simulink model "m03_linearization_model_4DOF"  (R2021a)
settings: Solver=VariableStepAuto  StartTime=0.0  StopTime=10  RelTol=1e-3
values from neighbouring files (symbols this model uses):
  a = L - b    (= 1.43208)    [m00_params.m]    (also in params.mat)
  b = distr*L/(1 + distr)    (= 1.62792)    [m00_params.m]    (also in params.mat)
  F_damper = [-2018 -1498 -1198 -898 -530 0 305 552 734 942 1306]    [damper.mat]    (also in m00_params.m = F_damper)
  Ff_spring = [-4676.870968 -4635.060192 -4593.2364576 -4551.3997648 -4509.5501136 -4467.687504 -4425.811936 -4383.9234096 -4342.0219248 -4300.1074816 -4258.18008 -4216.23972 ... (221 elements, 1x221)]    [spring.mat]
  Fr_spring = [-6174.79580863 -6119.36435311 -6063.92211228 -6008.46902741 -5953.00503974 -5897.53009054 -5842.04412106 -5786.54707256 -5731.0388863 -5675.51950353 -5619.98886552 -5564.44691352 ... (221 elements, 1x221)]    [spring.mat]
  FzF_0_w = FzF_0/2    (= 6523.65)    [m00_params.m]
  FzR_0_w = FzR_0/2    (= 5738.85)    [m00_params.m]
  h_CoG = 0.642    [m00_params.m]    (also in params.mat)
  h_RC = h_CoG - hs    (= 0.116)    [m00_params.m]    (also in params2.mat)
  hs = 0.526    [m00_params.m]
  hu = 0.4    [m00_params.m]    (also in params2.mat)
  Ix = 850    [m00_params.m]
  Iz = 4600    [m00_params.m]
  Kt = (Kt_f + Kt_r)/2    (= 306000)    [m00_params.m]
  M = 2500    [m00_params.m]    (also in params.mat)
  ms = M - mu    (= 2159)    [m00_params.m]
  mu = 2*(mui)    (= 341)    [m00_params.m]
  mui = mui_f + mui_r    (= 170.5)    [m00_params.m]
  tw = (tw_F + tw_R)/2    (= 1.6675)    [m00_params.m]
  v_damper = [-0.52 -0.26 -0.13 -0.05 -0.02 0 0.02 0.05 0.13 0.26 0.52]    [damper.mat]
  Z_spring = [-0.11 -0.109 -0.108 -0.107 -0.106 -0.105 -0.104 -0.103 -0.102 -0.101 -0.1 -0.099 ... (221 elements, 1x221)]    [spring.mat]
settings Model: Creator=jaime  LastModifiedBy=jaime

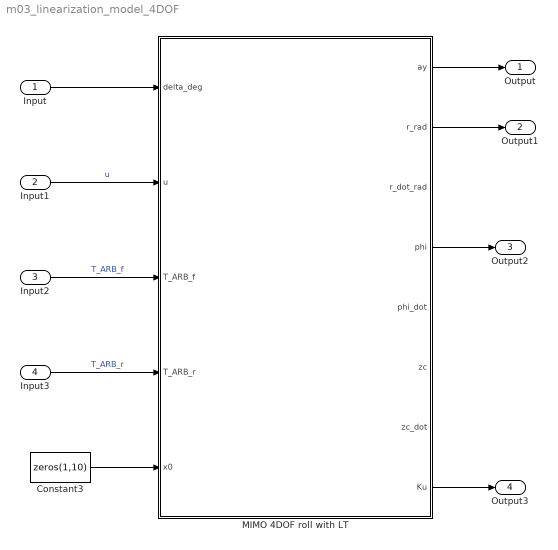
== system m03_linearization_model_4DOF ==
  Input : Inport
  Input1 : Inport  Port=2
  Input2 : Inport  Port=3
  Input3 : Inport  Port=4
  Constant3 : Constant  Value=zeros(1,10)
  MIMO 4DOF roll with LT : Subsystem
  Output : Outport
  Output1 : Outport  Port=2
  Output2 : Outport  Port=3
  Output3 : Outport  Port=4
  wires:
  Input1/1 -> MIMO 4DOF roll with LT/2(u)  "u"
  Input/1 -> MIMO 4DOF roll with LT/1(delta_deg)
  Input2/1 -> MIMO 4DOF roll with LT/3(T_ARB_f)  "T_ARB_f"
  Input3/1 -> MIMO 4DOF roll with LT/4(T_ARB_r)  "T_ARB_r"
  Constant3/1 -> MIMO 4DOF roll with LT/5(x0)
  MIMO 4DOF roll with LT/1(ay) -> Output/1
  MIMO 4DOF roll with LT/2(r_rad) -> Output1/1
  MIMO 4DOF roll with LT/4(phi) -> Output2/1
  MIMO 4DOF roll with LT/8(Ku) -> Output3/1

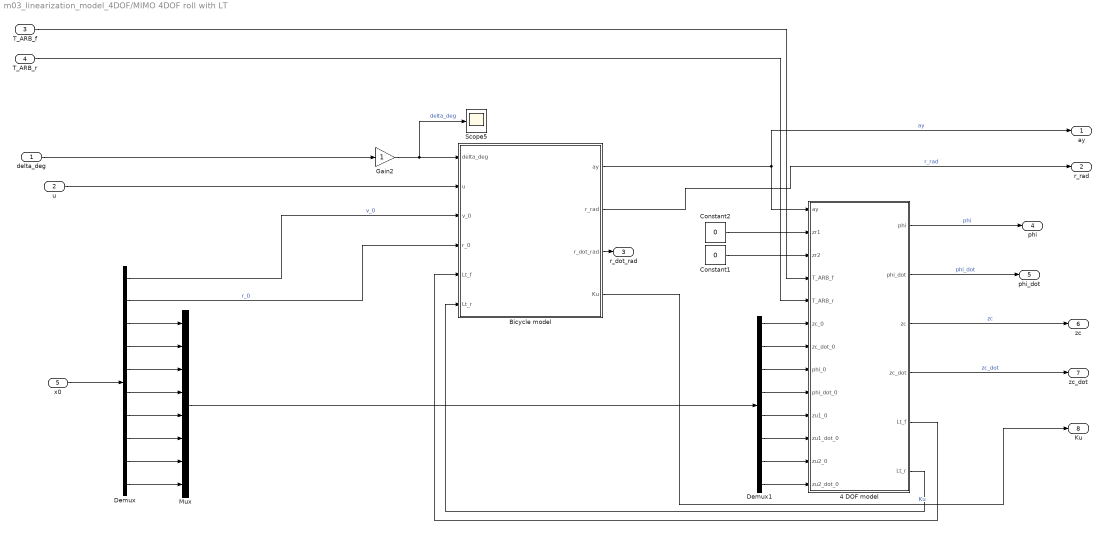
== system m03_linearization_model_4DOF/MIMO 4DOF roll with LT ==
  delta_deg : Inport
  u : Inport  Port=2
  T_ARB_f : Inport  Port=3
  T_ARB_r : Inport  Port=4
  x0 : Inport  Port=5
  4 DOF model : Subsystem
  Bicycle model : Subsystem
  Constant1 : Constant  Value=0
  Constant2 : Constant  Value=0
  Demux : Demux  Outputs=10
  Demux1 : Demux  Outputs=8
  Gain2 : Gain
  Mux : Mux  Inputs=8
  Scope5 : Scope
  ay : Outport
  r_rad : Outport  Port=2
  r_dot_rad : Outport  Port=3
  phi : Outport  Port=4
  phi_dot : Outport  Port=5
  zc : Outport  Port=6
  zc_dot : Outport  Port=7
  Ku : Outport  Port=8
  wires:
  Demux/10 -> Mux/8
  Demux1/6 -> 4 DOF model/11(zu1_dot_0)
  u/1 -> Bicycle model/2(u)
  Gain2/1 -> Scope5/1, Bicycle model/1(delta_deg)  "delta_deg"
  Demux/6 -> Mux/4
  Demux1/8 -> 4 DOF model/13(zu2_dot_0)
  4 DOF model/6(Lt_r) -> Bicycle model/6(Lt_r)
  Demux1/7 -> 4 DOF model/12(zu2_0)
  Demux1/5 -> 4 DOF model/10(zu1_0)
  Demux1/3 -> 4 DOF model/8(phi_0)
  Bicycle model/3(r_dot_rad) -> r_dot_rad/1
  T_ARB_r/1 -> 4 DOF model/5(T_ARB_r)
  Demux/9 -> Mux/7
  Constant1/1 -> 4 DOF model/3(zr2)
  Constant2/1 -> 4 DOF model/2(zr1)
  delta_deg/1 -> Gain2/1
  Bicycle model/1(ay) -> ay/1, 4 DOF model/1(ay)  "ay"
  Demux/3 -> Mux/1
  Demux/5 -> Mux/3
  Mux/1 -> Demux1/1
  Demux1/2 -> 4 DOF model/7(zc_dot_0)
  Demux/7 -> Mux/5
  Bicycle model/4(Ku) -> Ku/1  "Ku"
  4 DOF model/2(phi_dot) -> phi_dot/1  "phi_dot"
  4 DOF model/5(Lt_f) -> Bicycle model/5(Lt_f)
  Demux/4 -> Mux/2
  Demux1/1 -> 4 DOF model/6(zc_0)
  Demux1/4 -> 4 DOF model/9(phi_dot_0)
  Demux/2 -> Bicycle model/4(r_0)  "r_0"
  Demux/8 -> Mux/6
  Demux/1 -> Bicycle model/3(v_0)  "v_0"
  Bicycle model/2(r_rad) -> r_rad/1  "r_rad"
  x0/1 -> Demux/1
  4 DOF model/4(zc_dot) -> zc_dot/1  "zc_dot"
  T_ARB_f/1 -> 4 DOF model/4(T_ARB_f)
  4 DOF model/3(zc) -> zc/1  "zc"
  4 DOF model/1(phi) -> phi/1  "phi"

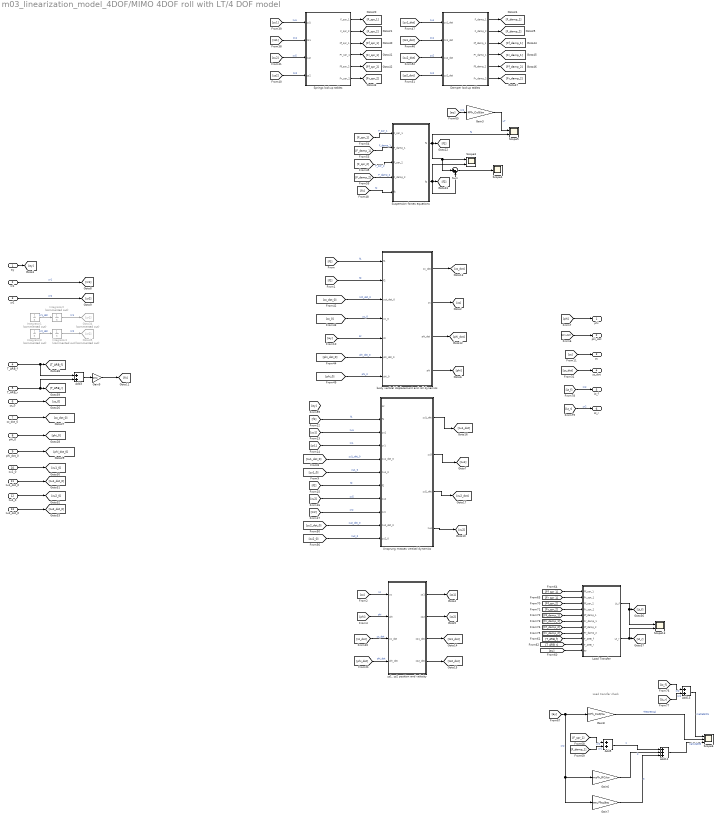
== system m03_linearization_model_4DOF/MIMO 4DOF roll with LT/4 DOF model ==
  note: Load transfer check
  ay : Inport
  zr1 : Inport  Port=2
  zr2 : Inport  Port=3
  T_ARB_f : Inport  Port=4
  T_ARB_r : Inport  Port=5
  zc_0 : Inport  Port=6
  zc_dot_0 : Inport  Port=7
  phi_0 : Inport  Port=8
  phi_dot_0 : Inport  Port=9
  zu1_0 : Inport  Port=10
  zu1_dot_0 : Inport  Port=11
  zu2_0 : Inport  Port=12
  zu2_dot_0 : Inport  Port=13
  Add12 : Sum  Inputs=+++
  Add13 : Sum
  Add3 : Sum
  Add5 : Sum
  Damper lookup tables : Subsystem
  Gain3 : Gain  Gain=M*h_CoG/tw
  Gain6 : Gain  Gain=ms*h_RC/tw
  Gain7 : Gain  Gain=mu*hu/tw
  Gain8 : Gain  Gain=M*h_CoG/tw
  Gain9 : Gain  Gain=1/tw
  Goto34 : Goto  Commented=on  GotoTag=zr1
  Goto35 : Goto  Commented=on  GotoTag=zr2
  Integrator{1..4} (4 alike) : Integrator  Commented=on
  Load Transfer : MATLAB Function  TreatAsAtomicUnit=on
  Scope13 : Scope  NumInputPorts=2
  Scope3 : Scope  NumInputPorts=2
  Scope4 : Scope
  Scope5 : Scope  NumInputPorts=2
  Scope6 : Scope  NumInputPorts=3
  Springs lookup tables : Subsystem
  Sum : Sum  Inputs=|++
  Suspension forces equations : Subsystem
  Unsprung masses vertical dynamics : Subsystem
  body vertical displacement and roll dynamics : Subsystem
  "zs1, zs2 position and velocity" : Subsystem
  phi : Outport
  phi_dot : Outport  Port=2
  zc : Outport  Port=3
  zc_dot : Outport  Port=4
  Lt_f : Outport  Port=5
  Lt_r : Outport  Port=6
  wires:
  [phi] -> phi/1
  ay/1 -> [ay]
  [zc] -> zc/1
  zr1/1 -> [zr1]  "zr1"
  zr2/1 -> [zr2]  "zr2"
  [phi_dot] -> phi_dot/1
  [zc_dot] -> zc_dot/1
  [zu1] -> Springs lookup tables/1(zu1)  "zu1"
  [zs1] -> Springs lookup tables/2(zs1)  "zs1"
  [zu2] -> Springs lookup tables/3(zu2)  "zu2"
  [zs2] -> Springs lookup tables/4(zs2)  "zs2"
  Springs lookup tables/1(F_spr_1) -> [F_spr_1]
  Springs lookup tables/2(F_spr_2) -> [F_spr_2]
  [zu1_dot] -> Damper lookup tables/1(zu1_dot)  "zu1"
  [zs2_dot] -> Damper lookup tables/4(zs2_dot)  "zs2"
  [zs1_dot] -> Damper lookup tables/2(zs1_dot)  "zs1"
  [zu2_dot] -> Damper lookup tables/3(zu2_dot)  "zu2"
  Damper lookup tables/1(F_damp_1) -> [F_damp_1]
  Damper lookup tables/2(F_damp_2) -> [F_damp_2]
  [F_spr_1] -> Suspension forces equations/1(F_spr_1)  "F_spr_1"
  [F_damp_1] -> Suspension forces equations/2(F_damp_1)  "F_damp_1"
  [F_spr_2] -> Suspension forces equations/3(F_spr_2)  "F_spr_2"
  [F_damp_2] -> Suspension forces equations/4(F_damp_2)  "F_damp_2"
  [fc] -> Suspension forces equations/5(fc)  "fc"
  Suspension forces equations/1(f1) -> Scope5/2, [f1], Sum/1, Scope3/1  "f1"
  Suspension forces equations/2(f2) -> Scope3/2, Sum/2, [f2]
  zc_0/1 -> [zc_0]
  zc_dot_0/1 -> [zc_dot_0]
  phi_dot_0/1 -> [phi_dot_0]
  phi_0/1 -> [phi_0]
  [f1] -> body vertical displacement and roll dynamics/1(f1)  "f1"
  [f2] -> body vertical displacement and roll dynamics/2(f2)  "f2"
  [zc_dot_0] -> body vertical displacement and roll dynamics/3(zct_dot_0)  "zct_dot_0"
  [zc_0] -> body vertical displacement and roll dynamics/4(zc_0)  "zc_0"
  [ay] -> body vertical displacement and roll dynamics/5(ay)  "ay"
  [phi_dot_0] -> body vertical displacement and roll dynamics/6(phi_dot_0)  "phi_dot_0"
  [phi_0] -> body vertical displacement and roll dynamics/7(phi_0)  "phi_0"
  body vertical displacement and roll dynamics/1(zc_dot) -> [zc_dot]
  body vertical displacement and roll dynamics/2(zc) -> [zc]
  body vertical displacement and roll dynamics/3(phi_dot) -> [phi_dot]
  body vertical displacement and roll dynamics/4(phi) -> [phi]
  zu1_0/1 -> [zu1_0]
  zu2_dot_0/1 -> [zu2_dot_0]
  zu2_0/1 -> [zu2_0]
  zu1_dot_0/1 -> [zu1_dot_0]
  [f1] -> Unsprung masses vertical dynamics/2(f1)  "f1"
  [zu1] -> Unsprung masses vertical dynamics/3(zu1)  "zu1"
  [zr1] -> Unsprung masses vertical dynamics/4(zr1)  "zr1"
  [zu1_dot_0] -> Unsprung masses vertical dynamics/5(zu1_dot_0)  "zu1_dot_0"
  [zu1_0] -> Unsprung masses vertical dynamics/6(zu1_0)  "zu1_0"
  [f2] -> Unsprung masses vertical dynamics/7(f2)  "f2"
  [zu2] -> Unsprung masses vertical dynamics/8(zu2)  "zu2"
  [zr2] -> Unsprung masses vertical dynamics/9(zr2)  "zr2"
  [zu2_dot_0] -> Unsprung masses vertical dynamics/10(zu2_dot_0)  "zu2_dot_0"
  [zu2_0] -> Unsprung masses vertical dynamics/11(zu2_0)  "zu2_0"
  Unsprung masses vertical dynamics/1(zu1_dot) -> [zu1_dot]
  Unsprung masses vertical dynamics/2(zu3) -> [zu1]
  Unsprung masses vertical dynamics/3(zu2_dot) -> [zu2_dot]
  Unsprung masses vertical dynamics/4(zu4) -> [zu2]
  [zc] -> "zs1, zs2 position and velocity"/1(zc)  "zc"
  [phi] -> "zs1, zs2 position and velocity"/2(phi)  "phi"
  [zc_dot] -> "zs1, zs2 position and velocity"/3(zc_dot)  "zc_dot"
  [phi_dot] -> "zs1, zs2 position and velocity"/4(phi_dot)  "phi_dot"
  "zs1, zs2 position and velocity"/1(zs1) -> [zs1]
  "zs1, zs2 position and velocity"/2(zs2) -> [zs2]
  "zs1, zs2 position and velocity"/3(zs1_dot) -> [zs1_dot]
  "zs1, zs2 position and velocity"/4(zs2_dot) -> [zs2_dot]
  Integrator2/1 -> Goto34/1  "zr1"
  Integrator4/1 -> Goto35/1  "zr2"
  Integrator3/1 -> Integrator4/1  "zr2_dot"
  Integrator1/1 -> Integrator2/1  "zr1_dot"
  Gain9/1 -> [fc]
  T_ARB_f/1 -> Add3/1, [T_ARB_f]
  T_ARB_r/1 -> Add3/2, [T_ARB_r]
  Add3/1 -> Gain9/1
  Sum/1 -> Scope4/1
  [ay] -> Gain3/1  "zr2"
  Gain3/1 -> Scope5/1  "LT"
  Springs lookup tables/3(Ff_spr_1) -> [Ff_spr_1]
  Springs lookup tables/4(Fr_spr_1) -> [Fr_spr_1]
  Springs lookup tables/5(Ff_spr_2) -> [Ff_spr_2]
  Springs lookup tables/6(Fr_spr_2) -> [Fr_spr_2]
  [F_spr_1] -> Add5/1  "zr2"
  [F_damp_1] -> Add5/2  "zr2"
  Add5/1 -> Add12/1  "1"
  [ay] -> Gain8/1, Gain7/1, Gain6/1  "zr2"
  Gain6/1 -> Add12/2  "2"
  Gain7/1 -> Add12/3  "3"
  Add12/1 -> Scope6/3  "calculated"
  Gain8/1 -> Scope6/2  "Theoretical"
  [Ff_spr_1] -> Load Transfer/1(Ff_spr_1)
  [T_ARB_r] -> Load Transfer/10(T_ARB_r)
  [Fr_spr_1] -> Load Transfer/2(Fr_spr_1)
  [T_ARB_f] -> Load Transfer/9(T_ARB_f)
  Load Transfer/1(Lt_f) -> Scope13/1, [Lt_f]
  [ay] -> Load Transfer/11(ay)
  Load Transfer/2(Lt_r) -> Scope13/2, [Lt_r]
  Damper lookup tables/3(Ff_damp_1) -> [Ff_damp_1]
  Damper lookup tables/4(Fr_damp_1) -> [Fr_damp_1]
  Damper lookup tables/5(Ff_damp_2) -> [Ff_damp_2]
  Damper lookup tables/6(Fr_damp_2) -> [Fr_damp_2]
  [Ff_spr_2] -> Load Transfer/3(Ff_spr_2)
  [Fr_spr_2] -> Load Transfer/4(Fr_spr_2)
  [Ff_damp_1] -> Load Transfer/5(Ff_damp_1)
  [Fr_damp_1] -> Load Transfer/6(Fr_damp_1)
  [Ff_damp_2] -> Load Transfer/7(Ff_damp_2)
  [Fr_damp_2] -> Load Transfer/8(Fr_damp_2)
  [Lt_f] -> Add13/1  "zr2"
  [Lt_r] -> Add13/2  "zr2"
  Add13/1 -> Scope6/1  "matlabFCN"
  [Lt_f] -> Lt_f/1  "zr2"
  [Lt_r] -> Lt_r/1  "zr2"

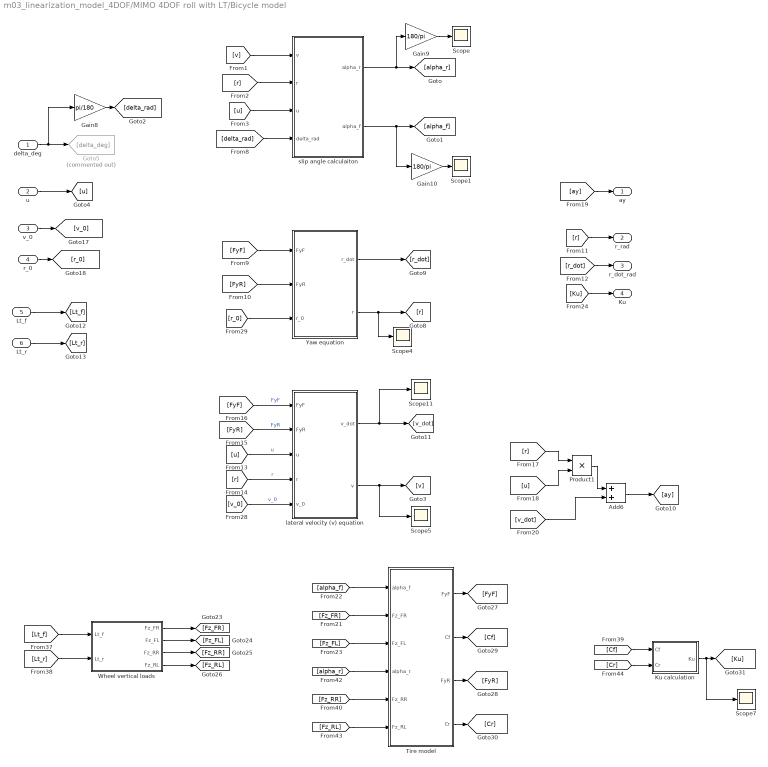
== system m03_linearization_model_4DOF/MIMO 4DOF roll with LT/Bicycle model ==
  delta_deg : Inport
  u : Inport  Port=2
  v_0 : Inport  Port=3
  r_0 : Inport  Port=4
  Lt_f : Inport  Port=5
  Lt_r : Inport  Port=6
  Add6 : Sum
  Gain10 : Gain  Gain=180/pi
  Gain8 : Gain  Gain=pi/180
  Gain9 : Gain  Gain=180/pi
  Goto5 : Goto  Commented=on  GotoTag=delta_deg
  Ku calculation : MATLAB Function  TreatAsAtomicUnit=on
  Product1 : Product
  Scope{,1,4..5,7,11} (6 alike) : Scope
  Tire model : Subsystem
      settings: AttributesFormatString=%<MinAlgLoopOccurrences>
  Wheel vertical loads : Subsystem
      settings: AttributesFormatString=%<MinAlgLoopOccurrences>
  Yaw equation : Subsystem
  lateral velocity (v) equation : Subsystem
  slip angle calculaiton : Subsystem
  ay : Outport
  r_rad : Outport  Port=2
  r_dot_rad : Outport  Port=3
  Ku : Outport  Port=4
  wires:
  u/1 -> [u]
  delta_deg/1 -> Gain8/1, Goto5/1
  [r] -> r_rad/1
  [r_dot] -> r_dot_rad/1
  [r] -> Product1/1
  [u] -> Product1/2
  [ay] -> ay/1
  Gain8/1 -> [delta_rad]
  Add6/1 -> [ay]
  Product1/1 -> Add6/1
  [v_dot] -> Add6/2
  Wheel vertical loads/4(Fz_RL) -> [Fz_RL]
  [Lt_f] -> Wheel vertical loads/1(Lt_f)
  [Lt_r] -> Wheel vertical loads/2(Lt_r)
  Wheel vertical loads/1(Fz_FR) -> [Fz_FR]
  Wheel vertical loads/3(Fz_RR) -> [Fz_RR]
  Wheel vertical loads/2(Fz_FL) -> [Fz_FL]
  Lt_f/1 -> [Lt_f]
  Lt_r/1 -> [Lt_r]
  [Fz_RR] -> Tire model/5(Fz_RR)
  Tire model/3(FyR) -> [FyR]
  Tire model/2(Cf) -> [Cf]
  Tire model/1(FyF) -> [FyF]
  [Fz_FL] -> Tire model/3(Fz_FL)
  [Fz_FR] -> Tire model/2(Fz_FR)
  [alpha_r] -> Tire model/4(alpha_r)
  Tire model/4(Cr) -> [Cr]
  [Fz_RL] -> Tire model/6(Fz_RL)
  [alpha_f] -> Tire model/1(alpha_f)
  [Cr] -> Ku calculation/2(Cr)
  [Cf] -> Ku calculation/1(Cf)
  Ku calculation/1(Ku) -> Scope7/1, [Ku]
  [Ku] -> Ku/1
  slip angle calculaiton/2(alpha_f) -> Gain10/1, [alpha_f]
  [r] -> slip angle calculaiton/2(r)
  [u] -> slip angle calculaiton/3(u)
  slip angle calculaiton/1(alpha_r) -> [alpha_r], Gain9/1
  Gain9/1 -> Scope/1
  [delta_rad] -> slip angle calculaiton/4(delta_rad)
  Gain10/1 -> Scope1/1
  [v] -> slip angle calculaiton/1(v)
  v_0/1 -> [v_0]
  r_0/1 -> [r_0]
  [r_0] -> Yaw equation/3(r_0)
  [FyR] -> Yaw equation/2(FyR)
  Yaw equation/1(r_dot) -> [r_dot]
  [FyF] -> Yaw equation/1(FyF)
  Yaw equation/2(r) -> [r], Scope4/1
  [FyR] -> lateral velocity (v) equation/2(FyR)  "FyR"
  [u] -> lateral velocity (v) equation/3(u)  "u"
  [FyF] -> lateral velocity (v) equation/1(FyF)  "FyF"
  [v_0] -> lateral velocity (v) equation/5(v_0)  "v_0"
  lateral velocity (v) equation/2(v) -> [v], Scope5/1
  lateral velocity (v) equation/1(v_dot) -> [v_dot], Scope11/1
  [r] -> lateral velocity (v) equation/4(r)  "r"

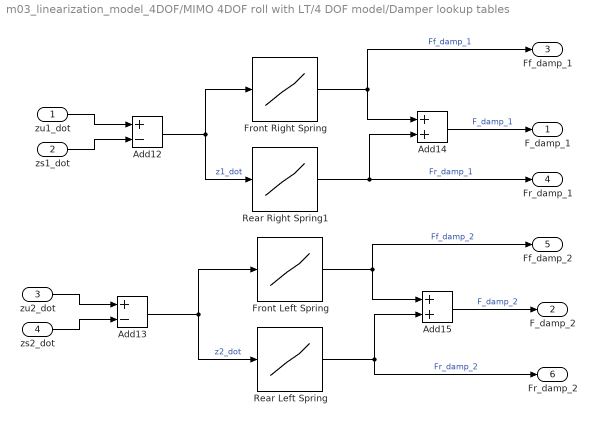
== system m03_linearization_model_4DOF/MIMO 4DOF roll with LT/4 DOF model/Damper lookup tables ==
  zu1_dot : Inport
  zs1_dot : Inport  Port=2
  zu2_dot : Inport  Port=3
  zs2_dot : Inport  Port=4
  Add12 : Sum  Inputs=+-
  Add13 : Sum  Inputs=+-
  Add14 : Sum
  Add15 : Sum
  Front Left Spring : Lookup_n-D  NumberOfTableDimensions=1  BreakpointsForDimension1=v_damper  Table=F_damper  InternalRulePriority=Speed  RndMeth=Simplest  InputSameDT=on
  Front Right Spring : Lookup_n-D  NumberOfTableDimensions=1  BreakpointsForDimension1=v_damper  Table=F_damper  InternalRulePriority=Speed  RndMeth=Simplest  InputSameDT=on
  Rear Left Spring : Lookup_n-D  NumberOfTableDimensions=1  BreakpointsForDimension1=v_damper  Table=F_damper  InternalRulePriority=Speed  RndMeth=Simplest  InputSameDT=on
  Rear Right Spring1 : Lookup_n-D  NumberOfTableDimensions=1  BreakpointsForDimension1=v_damper  Table=F_damper  InternalRulePriority=Speed  RndMeth=Simplest  InputSameDT=on
  F_damp_1 : Outport
  F_damp_2 : Outport  Port=2
  Ff_damp_1 : Outport  Port=3
  Fr_damp_1 : Outport  Port=4
  Ff_damp_2 : Outport  Port=5
  Fr_damp_2 : Outport  Port=6
  wires:
  zu1_dot/1 -> Add12/1
  Add13/1 -> Front Left Spring/1, Rear Left Spring/1  "z2_dot"
  Rear Right Spring1/1 -> Fr_damp_1/1, Add14/2  "Fr_damp_1"
  Add12/1 -> Rear Right Spring1/1, Front Right Spring/1  "z1_dot"
  Rear Left Spring/1 -> Fr_damp_2/1, Add15/2  "Fr_damp_2"
  Front Right Spring/1 -> Ff_damp_1/1, Add14/1  "Ff_damp_1"
  zu2_dot/1 -> Add13/1
  Front Left Spring/1 -> Add15/1, Ff_damp_2/1  "Ff_damp_2"
  zs2_dot/1 -> Add13/2
  zs1_dot/1 -> Add12/2
  Add14/1 -> F_damp_1/1  "F_damp_1"
  Add15/1 -> F_damp_2/1  "F_damp_2"

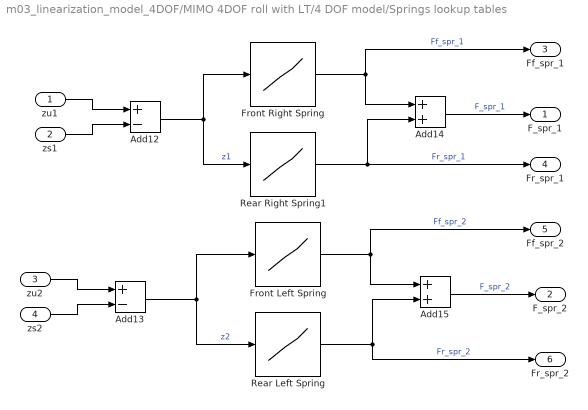
== system m03_linearization_model_4DOF/MIMO 4DOF roll with LT/4 DOF model/Springs lookup tables ==
  zu1 : Inport
  zs1 : Inport  Port=2
  zu2 : Inport  Port=3
  zs2 : Inport  Port=4
  Add12 : Sum  Inputs=+-
  Add13 : Sum  Inputs=+-
  Add14 : Sum
  Add15 : Sum
  Front Left Spring : Lookup_n-D  NumberOfTableDimensions=1  BreakpointsForDimension1=Z_spring  Table=Ff_spring  InternalRulePriority=Speed  RndMeth=Simplest  InputSameDT=on
  Front Right Spring : Lookup_n-D  NumberOfTableDimensions=1  BreakpointsForDimension1=Z_spring  Table=Ff_spring  InternalRulePriority=Speed  RndMeth=Simplest  InputSameDT=on
  Rear Left Spring : Lookup_n-D  NumberOfTableDimensions=1  BreakpointsForDimension1=Z_spring  Table=Fr_spring  InternalRulePriority=Speed  RndMeth=Simplest  InputSameDT=on
  Rear Right Spring1 : Lookup_n-D  NumberOfTableDimensions=1  BreakpointsForDimension1=Z_spring  Table=Fr_spring  InternalRulePriority=Speed  RndMeth=Simplest  InputSameDT=on
  F_spr_1 : Outport
  F_spr_2 : Outport  Port=2
  Ff_spr_1 : Outport  Port=3
  Fr_spr_1 : Outport  Port=4
  Ff_spr_2 : Outport  Port=5
  Fr_spr_2 : Outport  Port=6
  wires:
  zu1/1 -> Add12/1
  Add13/1 -> Front Left Spring/1, Rear Left Spring/1  "z2"
  Rear Right Spring1/1 -> Fr_spr_1/1, Add14/2  "Fr_spr_1"
  Add12/1 -> Rear Right Spring1/1, Front Right Spring/1  "z1"
  Rear Left Spring/1 -> Fr_spr_2/1, Add15/2  "Fr_spr_2"
  Front Right Spring/1 -> Add14/1, Ff_spr_1/1  "Ff_spr_1"
  zu2/1 -> Add13/1
  Front Left Spring/1 -> Ff_spr_2/1, Add15/1  "Ff_spr_2"
  zs2/1 -> Add13/2
  zs1/1 -> Add12/2
  Add14/1 -> F_spr_1/1  "F_spr_1"
  Add15/1 -> F_spr_2/1  "F_spr_2"

== system m03_linearization_model_4DOF/MIMO 4DOF roll with LT/4 DOF model/Suspension forces equations ==
  F_spr_1 : Inport
  F_damp_1 : Inport  Port=2
  F_spr_2 : Inport  Port=3
  F_damp_2 : Inport  Port=4
  fc : Inport  Port=5
  Add12 : Sum  Inputs=+++
  Add17 : Sum  Inputs=++-
  f1 : Outport
  f2 : Outport  Port=2
  wires:
  F_spr_2/1 -> Add17/1
  F_damp_1/1 -> Add12/2
  Add17/1 -> f2/1  "f2"
  fc/1 -> Add17/3, Add12/3
  F_spr_1/1 -> Add12/1
  Add12/1 -> f1/1  "f1"
  F_damp_2/1 -> Add17/2

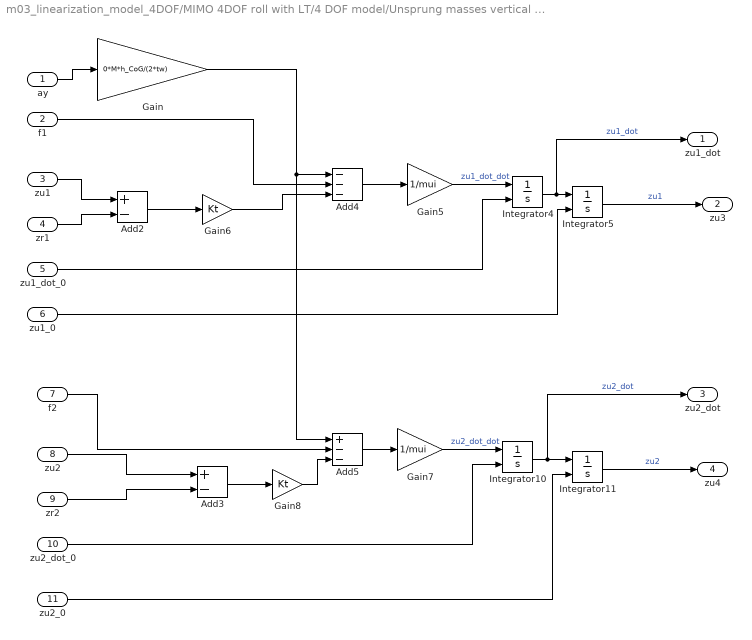
== system m03_linearization_model_4DOF/MIMO 4DOF roll with LT/4 DOF model/Unsprung masses vertical dynamics ==
  ay : Inport
  f1 : Inport  Port=2
  zu1 : Inport  Port=3
  zr1 : Inport  Port=4
  zu1_dot_0 : Inport  Port=5
  zu1_0 : Inport  Port=6
  f2 : Inport  Port=7
  zu2 : Inport  Port=8
  zr2 : Inport  Port=9
  zu2_dot_0 : Inport  Port=10
  zu2_0 : Inport  Port=11
  Add2 : Sum  Inputs=+-
  Add3 : Sum  Inputs=+-
  Add4 : Sum  Inputs=---
  Add5 : Sum  Inputs=+--
  Gain : Gain  Gain=0*M*h_CoG/(2*tw)
  Gain5 : Gain  Gain=1/mui
  Gain6 : Gain  Gain=Kt
  Gain7 : Gain  Gain=1/mui
  Gain8 : Gain  Gain=Kt
  Integrator{4..5,10..11} (4 alike) : Integrator  InitialConditionSource=external
  zu1_dot : Outport
  zu3 : Outport  Port=2
  zu2_dot : Outport  Port=3
  zu4 : Outport  Port=4
  wires:
  Integrator4/1 -> zu1_dot/1, Integrator5/1  "zu1_dot"
  Gain5/1 -> Integrator4/1  "zu1_dot_dot"
  Integrator5/1 -> zu3/1  "zu1"
  Add2/1 -> Gain6/1
  Add3/1 -> Gain8/1
  zu1_0/1 -> Integrator5/2
  Integrator10/1 -> zu2_dot/1, Integrator11/1  "zu2_dot"
  Add5/1 -> Gain7/1
  Gain8/1 -> Add5/3
  zu1/1 -> Add2/1
  Gain6/1 -> Add4/3
  Add4/1 -> Gain5/1
  Gain7/1 -> Integrator10/1  "zu2_dot_dot"
  zu2_0/1 -> Integrator11/2
  Integrator11/1 -> zu4/1  "zu2"
  zr2/1 -> Add3/2
  zu2/1 -> Add3/1
  zu2_dot_0/1 -> Integrator10/2
  f2/1 -> Add5/2
  zr1/1 -> Add2/2
  f1/1 -> Add4/2
  zu1_dot_0/1 -> Integrator4/2
  ay/1 -> Gain/1
  Gain/1 -> Add5/1, Add4/1

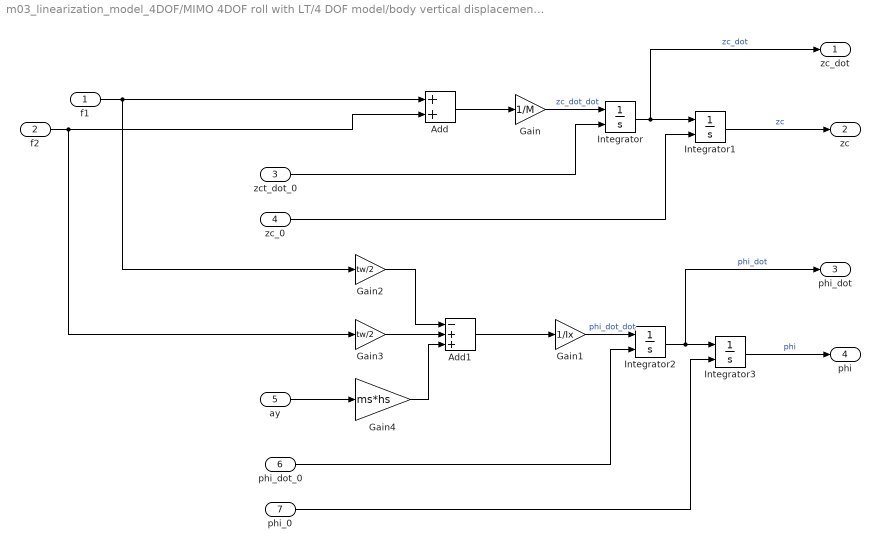
== system m03_linearization_model_4DOF/MIMO 4DOF roll with LT/4 DOF model/body vertical displacement and roll dynamics ==
  f1 : Inport
  f2 : Inport  Port=2
  zct_dot_0 : Inport  Port=3
  zc_0 : Inport  Port=4
  ay : Inport  Port=5
  phi_dot_0 : Inport  Port=6
  phi_0 : Inport  Port=7
  Add : Sum
  Add1 : Sum  Inputs=-++
  Gain : Gain  Gain=1/M
  Gain1 : Gain  Gain=1/Ix
  Gain2 : Gain  Gain=tw/2
  Gain3 : Gain  Gain=tw/2
  Gain4 : Gain  Gain=ms*hs
  Integrator{,1..3} (4 alike) : Integrator  InitialConditionSource=external
  zc_dot : Outport
  zc : Outport  Port=2
  phi_dot : Outport  Port=3
  phi : Outport  Port=4
  wires:
  Integrator2/1 -> phi_dot/1, Integrator3/1  "phi_dot"
  zct_dot_0/1 -> Integrator/2
  Gain3/1 -> Add1/2
  Integrator3/1 -> phi/1  "phi"
  Add/1 -> Gain/1
  Gain1/1 -> Integrator2/1  "phi_dot_dot"
  Gain/1 -> Integrator/1  "zc_dot_dot"
  Add1/1 -> Gain1/1
  ay/1 -> Gain4/1
  phi_0/1 -> Integrator3/2
  Gain2/1 -> Add1/1
  Gain4/1 -> Add1/3
  Integrator/1 -> zc_dot/1, Integrator1/1  "zc_dot"
  f1/1 -> Gain2/1, Add/1
  f2/1 -> Gain3/1, Add/2
  Integrator1/1 -> zc/1  "zc"
  phi_dot_0/1 -> Integrator2/2
  zc_0/1 -> Integrator1/2

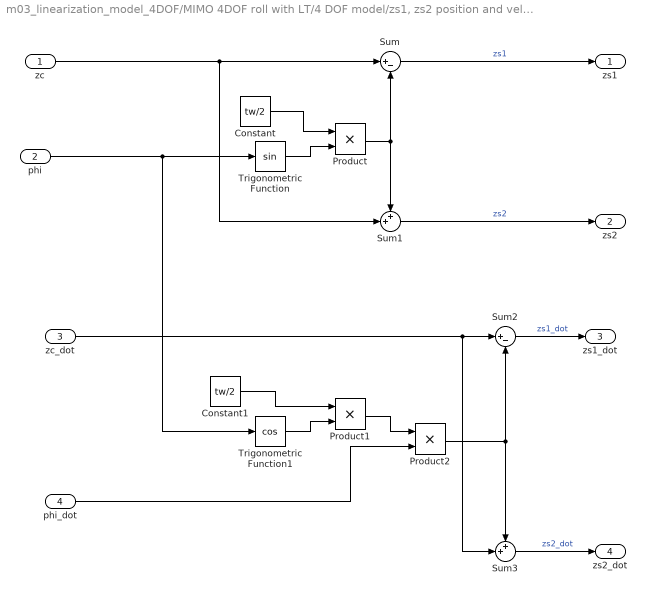
== system m03_linearization_model_4DOF/MIMO 4DOF roll with LT/4 DOF model/zs1, zs2 position and velocity ==
  zc : Inport
  phi : Inport  Port=2
  zc_dot : Inport  Port=3
  phi_dot : Inport  Port=4
  Constant : Constant  Value=tw/2
  Constant1 : Constant  Value=tw/2
  Product : Product
  Product1 : Product
  Product2 : Product
  Sum : Sum  Inputs=|+-
  Sum1 : Sum  Inputs=++|
  Sum2 : Sum  Inputs=|+-
  Sum3 : Sum  Inputs=++|
  Trigonometric Function : Trigonometry
  Trigonometric Function1 : Trigonometry  Operator=cos
  zs1 : Outport
  zs2 : Outport  Port=2
  zs1_dot : Outport  Port=3
  zs2_dot : Outport  Port=4
  wires:
  Product/1 -> Sum1/1, Sum/2
  Trigonometric Function/1 -> Product/2
  zc_dot/1 -> Sum3/2, Sum2/1
  Product1/1 -> Product2/1
  zc/1 -> Sum1/2, Sum/1
  Constant/1 -> Product/1
  Product2/1 -> Sum3/1, Sum2/2
  phi/1 -> Trigonometric Function1/1, Trigonometric Function/1
  Trigonometric Function1/1 -> Product1/2
  Constant1/1 -> Product1/1
  Sum/1 -> zs1/1  "zs1"
  Sum1/1 -> zs2/1  "zs2"
  Sum2/1 -> zs1_dot/1  "zs1_dot"
  Sum3/1 -> zs2_dot/1  "zs2_dot"
  phi_dot/1 -> Product2/2

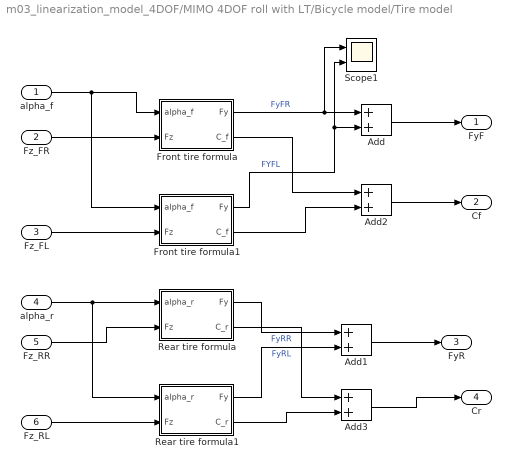
== system m03_linearization_model_4DOF/MIMO 4DOF roll with LT/Bicycle model/Tire model ==
  alpha_f : Inport
  Fz_FR : Inport  Port=2
  Fz_FL : Inport  Port=3
  alpha_r : Inport  Port=4
  Fz_RR : Inport  Port=5
  Fz_RL : Inport  Port=6
  Add{,1..3} (4 alike) : Sum
  Front tire formula : MATLAB Function  TreatAsAtomicUnit=on
      settings: AttributesFormatString=%<MinAlgLoopOccurrences>  MinAlgLoopOccurrences=on
  Front tire formula1 : MATLAB Function  TreatAsAtomicUnit=on
      settings: MinAlgLoopOccurrences=on
  Rear tire formula : MATLAB Function  TreatAsAtomicUnit=on
      settings: MinAlgLoopOccurrences=on
  Rear tire formula1 : MATLAB Function  TreatAsAtomicUnit=on
      settings: MinAlgLoopOccurrences=on
  Scope1 : Scope  NumInputPorts=2
  FyF : Outport
  Cf : Outport  Port=2
  FyR : Outport  Port=3
  Cr : Outport  Port=4
  wires:
  Rear tire formula/1(Fy) -> Add1/1  "FyRR"
  Fz_RL/1 -> Rear tire formula1/2(Fz)
  Fz_RR/1 -> Rear tire formula/2(Fz)
  Rear tire formula1/1(Fy) -> Add1/2  "FyRL"
  Fz_FR/1 -> Front tire formula/2(Fz)
  Fz_FL/1 -> Front tire formula1/2(Fz)
  alpha_f/1 -> Front tire formula1/1(alpha_f), Front tire formula/1(alpha_f)
  alpha_r/1 -> Rear tire formula1/1(alpha_r), Rear tire formula/1(alpha_r)
  Front tire formula/1(Fy) -> Scope1/1, Add/1  "FyFR"
  Front tire formula1/1(Fy) -> Scope1/2, Add/2  "FYFL"
  Add/1 -> FyF/1
  Add1/1 -> FyR/1
  Front tire formula/2(C_f) -> Add2/1
  Front tire formula1/2(C_f) -> Add2/2
  Add2/1 -> Cf/1
  Rear tire formula/2(C_r) -> Add3/1
  Rear tire formula1/2(C_r) -> Add3/2
  Add3/1 -> Cr/1

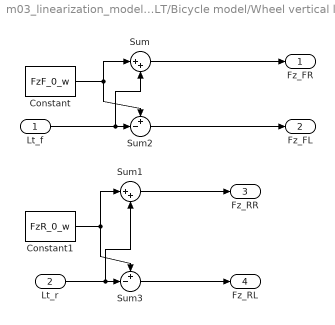
== system m03_linearization_model_4DOF/MIMO 4DOF roll with LT/Bicycle model/Wheel vertical loads ==
  Lt_f : Inport
  Lt_r : Inport  Port=2
  Constant : Constant  Value=FzF_0_w
  Constant1 : Constant  Value=FzR_0_w
  Sum : Sum  Inputs=|++
  Sum1 : Sum  Inputs=|++
  Sum2 : Sum  Inputs=+-|
  Sum3 : Sum  Inputs=+-|
  Fz_FR : Outport
  Fz_FL : Outport  Port=2
  Fz_RR : Outport  Port=3
  Fz_RL : Outport  Port=4
  wires:
  Constant/1 -> Sum2/1, Sum/1
  Constant1/1 -> Sum1/1, Sum3/1
  Sum1/1 -> Fz_RR/1
  Lt_f/1 -> Sum/2, Sum2/2
  Sum/1 -> Fz_FR/1
  Sum2/1 -> Fz_FL/1
  Lt_r/1 -> Sum1/2, Sum3/2
  Sum3/1 -> Fz_RL/1

== system m03_linearization_model_4DOF/MIMO 4DOF roll with LT/Bicycle model/Yaw equation ==
  FyF : Inport
  FyR : Inport  Port=2
  r_0 : Inport  Port=3
  Add3 : Sum  Inputs=+-
  Gain4 : Gain  Gain=1/Iz
  Gain5 : Gain  Gain=a
  Gain6 : Gain  Gain=b
  Integrator : Integrator  InitialConditionSource=external
  r_dot : Outport
  r : Outport  Port=2
  wires:
  Gain4/1 -> r_dot/1, Integrator/1  "r_dot"
  FyF/1 -> Gain5/1
  r_0/1 -> Integrator/2
  Gain5/1 -> Add3/1
  Gain6/1 -> Add3/2
  Add3/1 -> Gain4/1
  FyR/1 -> Gain6/1
  Integrator/1 -> r/1  "r"

== system m03_linearization_model_4DOF/MIMO 4DOF roll with LT/Bicycle model/lateral velocity (v) equation ==
  FyF : Inport
  FyR : Inport  Port=2
  u : Inport  Port=3
  r : Inport  Port=4
  v_0 : Inport  Port=5
  Add4 : Sum  Inputs=+-
  Add5 : Sum
  Gain7 : Gain  Gain=1/M
  Integrator1 : Integrator  InitialConditionSource=external
  Product : Product
  v_dot : Outport
  v : Outport  Port=2
  wires:
  Add4/1 -> v_dot/1, Integrator1/1  "v_dot"
  FyF/1 -> Add5/1
  Product/1 -> Add4/2
  Gain7/1 -> Add4/1
  Add5/1 -> Gain7/1
  Integrator1/1 -> v/1  "v"
  r/1 -> Product/2
  u/1 -> Product/1
  FyR/1 -> Add5/2
  v_0/1 -> Integrator1/2

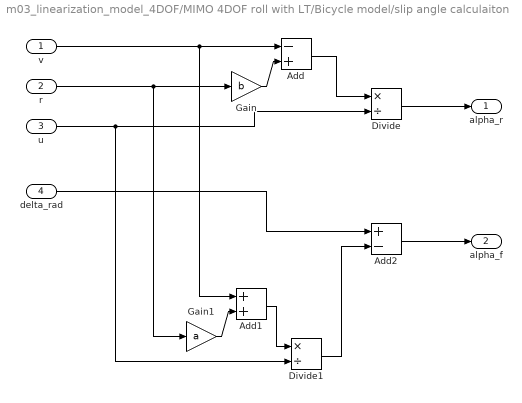
== system m03_linearization_model_4DOF/MIMO 4DOF roll with LT/Bicycle model/slip angle calculaiton ==
  v : Inport
  r : Inport  Port=2
  u : Inport  Port=3
  delta_rad : Inport  Port=4
  Add : Sum  Inputs=-+
  Add1 : Sum
  Add2 : Sum  Inputs=+-
  Divide : Product  Inputs=*/
  Divide1 : Product  Inputs=*/
  Gain : Gain  Gain=b
  Gain1 : Gain  Gain=a
  alpha_r : Outport
  alpha_f : Outport  Port=2
  wires:
  Gain1/1 -> Add1/2
  Divide1/1 -> Add2/2
  Add/1 -> Divide/1
  Add1/1 -> Divide1/1
  delta_rad/1 -> Add2/1
  r/1 -> Gain1/1, Gain/1
  Gain/1 -> Add/2
  Add2/1 -> alpha_f/1
  v/1 -> Add1/1, Add/1
  Divide/1 -> alpha_r/1
  u/1 -> Divide1/2, Divide/2

== matlab function m03_linearization_model_4DOF/MIMO 4DOF roll with LT/Bicycle model/Tire model/Front tire formula ==
  data: alpha_f input; Fy output; Fz input; C_f output
function [Fy, C_f] = fcn(alpha_f, Fz)
%% Pajecka formula for the front axle

mu_peak = 1.37 - Fz*0.026/1000;
mu_90_deg_f = 0.723*mu_peak;

Bf = 13; %% stiffness factor. Gives maximum mu for alpha = 6º for the static front tyre load.
Cf = 1.515; % Makes mu_max/mu_90_deg=0.723 for static front tyre load
Df = mu_peak; %% peak value. If Df<Dr understeer
Ef = Fz*(0.5+2)/12000 - 2; %% Curvature factor. Linear variation from Fz = 0KN to 12KN

mu_y_f = Df.*sin(Cf.*atan(Bf*alpha_f - Ef*(Bf*alpha_f - atan(Bf*alpha_f))));

n_f = (Cf.*Df.*cos(Cf.*atan(Bf.*alpha_f + Ef.*(atan(Bf.*alpha_f) - Bf.*alpha_f))).*(Bf - Ef.*(Bf - Bf./(Bf.^2.*alpha_f.^2 + 1))))./((Bf.*alpha_f + Ef.*(atan(Bf.*alpha_f) - Bf.*alpha_f)).^2 + 1);
C_f = n_f.*Fz;

Fy = mu_y_f*Fz;

% Fy = alpha;

== matlab function m03_linearization_model_4DOF/MIMO 4DOF roll with LT/4 DOF model/Load Transfer ==
  data: Ff_spr_1 input; Lt_f output; Lt_r output; Fr_spr_1 input; Ff_spr_2 input; Fr_spr_2 input; Ff_damp_1 input; Fr_damp_1 input; Ff_damp_2 input; Fr_damp_2 input; T_ARB_f input; T_ARB_r input; ay input
function [Lt_f, Lt_r] = fcn(Ff_spr_1, Fr_spr_1, Ff_spr_2, Fr_spr_2, Ff_damp_1, Fr_damp_1, Ff_damp_2, Fr_damp_2, T_ARB_f, T_ARB_r, ay)


St = load('params.mat');
St2 = load('params2.mat');
tw = 0.5*(St.tw_F + St.tw_R);

%% Load transfer in the front
Ltf_1 = ((Ff_spr_1 + Ff_damp_1) - (Ff_spr_2 + Ff_damp_2))/2 + T_ARB_f/St.tw_F; %% Load transfer due to roll (front)
Ltf_2 = St.ms_f*ay*St2.h_RC/St.tw_F;
Ltf_3 = St.mu_f*ay*St2.hu/St.tw_F;

Lt_f = Ltf_1 + Ltf_2 + Ltf_3;

%% Load transfer in the rear
Ltr_1 = ((Fr_spr_1 + Fr_damp_1) - (Fr_spr_2 + Fr_damp_2))/2 + T_ARB_r/St.tw_R; %% Load transfer due to roll (rear)
Ltr_2 = St.ms_r*ay*St2.h_RC/St.tw_R;
Ltr_3 = St.mu_r*ay*St2.hu/St.tw_R;

Lt_r = Ltr_1 + Ltr_2 + Ltr_3;

== matlab function m03_linearization_model_4DOF/MIMO 4DOF roll with LT/Bicycle model/Tire model/Front tire formula1 ==
  data: alpha_f input; Fy output; Fz input; C_f output
function [Fy, C_f] = fcn(alpha_f, Fz)
%% Pajecka formula for the front axle

mu_peak = 1.37 - Fz*0.026/1000;
mu_90_deg_f = 0.723*mu_peak;

Bf = 13; %% stiffness factor. Gives maximum mu for alpha = 6º for the static front tyre load.
Cf = 1.515; % Makes mu_max/mu_90_deg=0.723 for static front tyre load
Df = mu_peak; %% peak value. If Df<Dr understeer
Ef = Fz*(0.5+2)/12000 - 2; %% Curvature factor. Linear variation from Fz = 0KN to 12KN

mu_y_f = Df.*sin(Cf.*atan(Bf*alpha_f - Ef*(Bf*alpha_f - atan(Bf*alpha_f))));

n_f = (Cf.*Df.*cos(Cf.*atan(Bf.*alpha_f + Ef.*(atan(Bf.*alpha_f) - Bf.*alpha_f))).*(Bf - Ef.*(Bf - Bf./(Bf.^2.*alpha_f.^2 + 1))))./((Bf.*alpha_f + Ef.*(atan(Bf.*alpha_f) - Bf.*alpha_f)).^2 + 1);
C_f = n_f.*Fz;

Fy = mu_y_f*Fz;

% Fy = alpha;

== matlab function m03_linearization_model_4DOF/MIMO 4DOF roll with LT/Bicycle model/Tire model/Rear tire formula ==
  data: alpha_r input; Fy output; Fz input; C_r output
function [Fy, C_r] = fcn(alpha_r, Fz)
%% Pajecka formula for the front axle

mu_peak_r = 1.38 - Fz*0.0232/1000;
mu_90_deg_r = 0.723*mu_peak_r;

Br = 13; %% stiffness factor. Gives maximum mu for alpha = 6º for the static front tyre load.
Cr = 1.51253; % Makes mu_max/mu_90_deg=0.723 for static front tyre load
Dr = mu_peak_r; %% peak value. If Df<Dr understeer
Er = Fz*(0.5+2)/12000 - 2; %% Curvature factor. Linear variation from Fz = 0KN to 12KN

mu_y_r = Dr.*sin(Cr.*atan(Br*alpha_r - Er*(Br*alpha_r - atan(Br*alpha_r))));
n_r = (Cr.*Dr.*cos(Cr.*atan(Br.*alpha_r + Er.*(atan(Br.*alpha_r) - Br.*alpha_r))).*(Br - Er.*(Br - Br./(Br.^2.*alpha_r.^2 + 1))))./((Br.*alpha_r + Er.*(atan(Br.*alpha_r) - Br.*alpha_r)).^2 + 1);
C_r = n_r.*Fz;

Fy = mu_y_r*Fz;

% Fy = alpha;

== matlab function m03_linearization_model_4DOF/MIMO 4DOF roll with LT/Bicycle model/Tire model/Rear tire formula1 ==
  data: alpha_r input; Fy output; Fz input; C_r output
function [Fy, C_r] = fcn(alpha_r, Fz)
%% Pajecka formula for the front axle

mu_peak_r = 1.38 - Fz*0.0232/1000;
mu_90_deg_r = 0.723*mu_peak_r;

Br = 13; %% stiffness factor. Gives maximum mu for alpha = 6º for the static front tyre load.
Cr = 1.51253; % Makes mu_max/mu_90_deg=0.723 for static front tyre load
Dr = mu_peak_r; %% peak value. If Df<Dr understeer
Er = Fz*(0.5+2)/12000 - 2; %% Curvature factor. Linear variation from Fz = 0KN to 12KN

mu_y_r = Dr.*sin(Cr.*atan(Br*alpha_r - Er*(Br*alpha_r - atan(Br*alpha_r))));
n_r = (Cr.*Dr.*cos(Cr.*atan(Br.*alpha_r + Er.*(atan(Br.*alpha_r) - Br.*alpha_r))).*(Br - Er.*(Br - Br./(Br.^2.*alpha_r.^2 + 1))))./((Br.*alpha_r + Er.*(atan(Br.*alpha_r) - Br.*alpha_r)).^2 + 1);
C_r = n_r.*Fz;

Fy = mu_y_r*Fz;

% Fy = alpha;

== matlab function m03_linearization_model_4DOF/MIMO 4DOF roll with LT/Bicycle model/Ku calculation ==
  data: Cf input; Ku output; Cr input
function Ku = fcn(Cf, Cr)

S = load('params.mat');

Ku = S.M/S.L*((S.b*Cr - S.a*Cf)/(Cf*Cr));
